simulink model "conrolo_lqr"  (R2021b)
settings: Solver=VariableStepAuto  StartTime=0.0  StopTime=15.0  RelTol=1e-3
values from neighbouring files (symbols this model uses):
  A = [ ... (first row only)    [script.m]
  B = [ ... (first row only)    [script.m]
  C = [ ... (first row only)    [script.m]
  D = [ ... (first row only)    [script.m]
  h = 0.03    [script.m]
  L1 = dlqr(phi,gama,Q1,Q2)    [script.m]
  qi = [-0.17453 0 0 0]    [script.m]
settings Model: Creator=Dylan  LastModifiedBy=Dylan

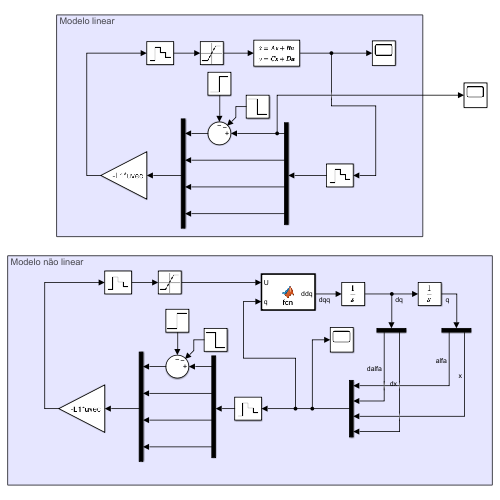
[thumbnail: Simulink's stored preview of the top-level diagram]
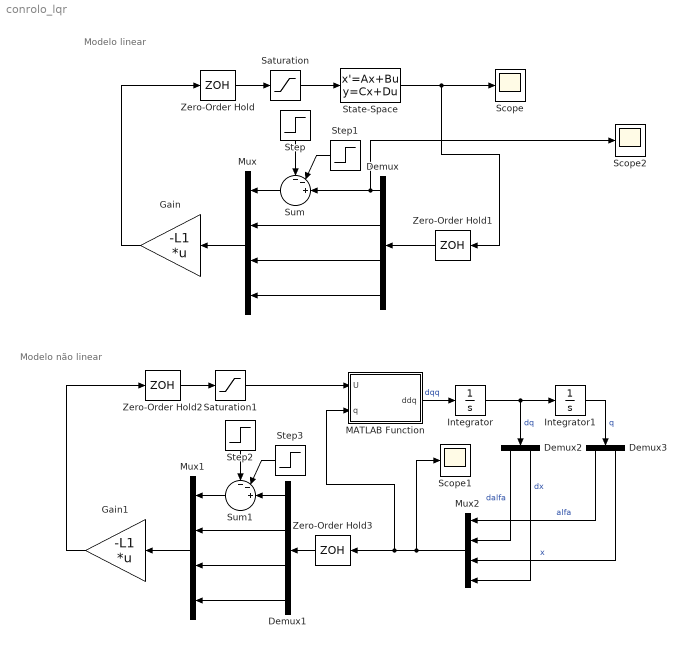
== system conrolo_lqr ==
  note: Modelo não linear
  note: Modelo linear
  Demux : Demux
  Demux1 : Demux
  Demux2 : Demux  Outputs=2
  Demux3 : Demux  Outputs=2
  Gain : Gain  Gain=-L1  Multiplication=Matrix(K*u) (u vector)
  Gain1 : Gain  Gain=-L1  Multiplication=Matrix(K*u) (u vector)
  Integrator : Integrator  InitialCondition=qi([2,4])
  Integrator1 : Integrator  InitialCondition=qi([1,3])
  MATLAB Function : MATLAB Function  TreatAsAtomicUnit=on
  Mux : Mux
  Mux1 : Mux
  Mux2 : Mux
  Saturation : Saturate  UpperLimit=4.8  LowerLimit=-4.8
  Saturation1 : Saturate  UpperLimit=4.8  LowerLimit=-4.8
  Scope : Scope
  Scope1 : Scope
  Scope2 : Scope
  State-Space : StateSpace  A=A  B=B  C=C  D=D  InitialCondition=qi
  Step : Step  Time=2  After=deg2rad(10)  SampleTime=0
  Step1 : Step  Time=8  After=-deg2rad(10)  SampleTime=0
  Step2 : Step  Time=2  After=deg2rad(10)  SampleTime=0
  Step3 : Step  Time=8  After=-deg2rad(10)  SampleTime=0
  Sum : Sum  Inputs=--+||
  Sum1 : Sum  Inputs=--+||
  Zero-Order Hold{,1..3} (4 alike) : ZeroOrderHold  SampleTime=h
  wires:
  Saturation/1 -> State-Space/1
  Zero-Order Hold/1 -> Saturation/1
  State-Space/1 -> Scope/1, Zero-Order Hold1/1
  Demux/2 -> Mux/2
  Demux/3 -> Mux/3
  Demux/4 -> Mux/4
  Zero-Order Hold1/1 -> Demux/1
  Mux/1 -> Gain/1
  Gain/1 -> Zero-Order Hold/1
  Sum/1 -> Mux/1
  Step/1 -> Sum/1
  Step1/1 -> Sum/2
  Zero-Order Hold2/1 -> Saturation1/1
  Gain1/1 -> Zero-Order Hold2/1
  Saturation1/1 -> MATLAB Function/1(U)
  Sum1/1 -> Mux1/1
  Demux1/4 -> Mux1/4
  Demux1/1 -> Sum1/3
  Step3/1 -> Sum1/2
  Demux1/2 -> Mux1/2
  Mux1/1 -> Gain1/1
  Step2/1 -> Sum1/1
  Demux1/3 -> Mux1/3
  MATLAB Function/1(ddq) -> Integrator/1  "dqq"
  Zero-Order Hold3/1 -> Demux1/1
  Integrator/1 -> Integrator1/1, Demux2/1  "dq"
  Integrator1/1 -> Demux3/1  "q"
  Mux2/1 -> Scope1/1, MATLAB Function/2(q), Zero-Order Hold3/1
  Demux3/1 -> Mux2/1  "alfa"
  Demux3/2 -> Mux2/3  "x"
  Demux2/1 -> Mux2/2  "dalfa"
  Demux2/2 -> Mux2/4  "dx"
  Demux/1 -> Sum/3, Scope2/1

== matlab function conrolo_lqr/MATLAB Function ==
  data: U input; ddq output; q input
function ddq = fcn(U,q)
Rm = 14;
Kb = 0.1343;
Kt = 0.0948;
L = 0.045;
Mp = 0.296;
Mw = 0.032;
Rw = 0.022;
lp = 0;
lw = 0.5*Mw*Rw^2;
g = 9.81;
h = 0.03;

alfa = q(1);
dalfa = q(2);
x = q(3);
dx= q(4);

% dq = [ddalfa; ddx]
% q = [da;dalfa]
% A * dq = B*U + C*q + D
% dq = inv(A)* (B*U + C*q + D)

A = [
    (lp+L^2*Mp) L*cos(alfa)*Mp
    L*cos(alfa)*Mp*Rw (lw/Rw + Mp*Rw+Mw*Rw)
];
B = [
  -Kt/Rm
  Kt/Rm
];
C = [
  (Kb*Kt)/(Rm*Rw) -(Kb*Kt)/Rm
  -(Kb*Kt)/(Rm*Rw) (Kb*Kt)/Rm
];
D = [
    g*L*sin(alfa)*Mp
    0
];
ddq = inv(A)*(B.*U + C*[dx;dalfa] + D);
